simulink model "defaultCtrlModel"  (R2022a)
settings: Solver=FixedStepAuto  StartTime=0.0  StopTime=1800  FixedStep=Ts  RelTol=1e-3
values from neighbouring files (symbols this model uses):
  Kt = 0.882355004501468    (= 0.882355004501)    [initModels_GUI.m]
  N = 3.75    [compareAdmittance.m]    (also in initModels_GUI.m)
libraries: simulink x2
settings Model: Creator=Johannes  LastModifiedBy=Johannes
settings SolverCC: ConcurrentTasks=on  AlgebraicLoopSolver=TrustRegion  PositivePriorityOrder=on
settings OptimizationCC: BlockReduction=off  OptimizeBlockIOStorage=off  ZeroExternalMemoryAtStartup=off  ZeroInternalMemoryAtStartup=off
settings DebuggingCC: TasksWithSamePriorityMsg=none  UnconnectedInputMsg=warning  UnconnectedOutputMsg=warning  UnconnectedLineMsg=warning  SFMachineParentedDataDiag=warning
settings HardwareCC: ProdBitPerLong=64  ProdLongLongMode=on  ProdHWDeviceType=Intel->x86-64 (Linux 64)
settings RTWCC: Description=Generic Real-Time Target  Toolchain=Simulink Real-Time Toolchain  BuildConfiguration=Faster Runs  TargetLang=C++  DLArmComputeVersion=19.05
settings GRTTargetCC: TargetLangStandard=C++03 (ISO)  CodeInterfacePackaging=C++ class

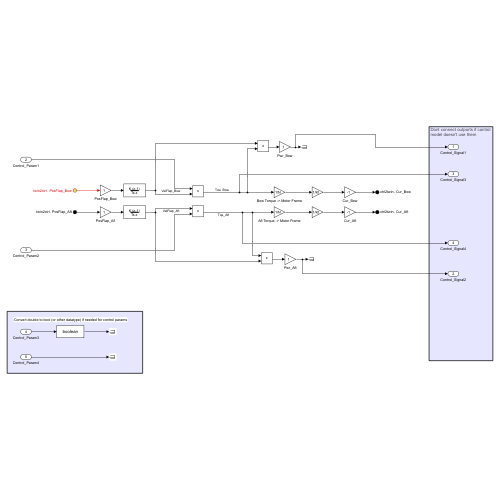
[thumbnail: Simulink's stored preview of the top-level diagram]
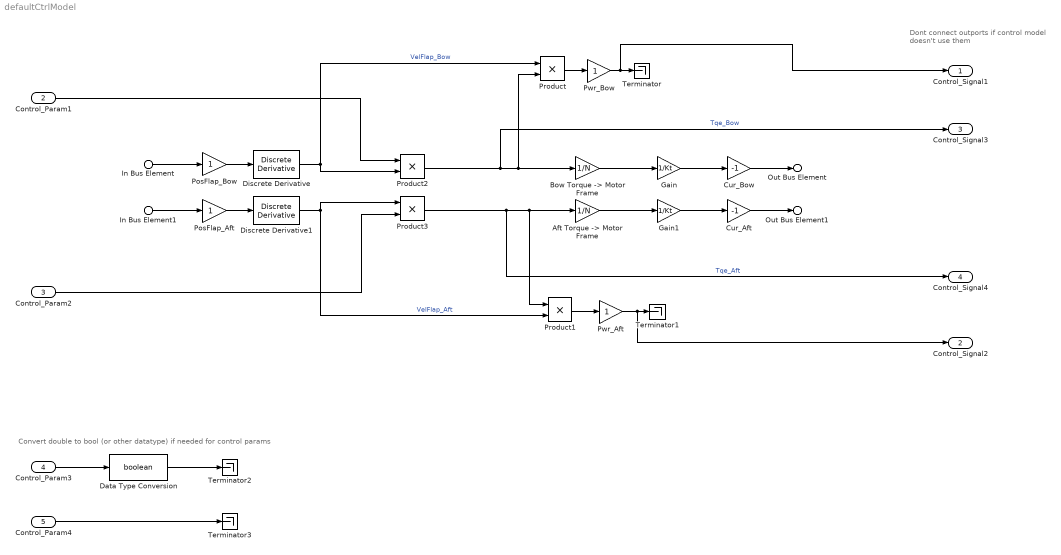
== system defaultCtrlModel ==
  note: Dont connect outports if control
      | model doesn't use them
  note: Convert double to bool (or other datatype) if needed for control params
  In Bus Element : Inport  PortName=twin2ctrl  Element=PosFlap_Bow
  In Bus Element1 : Inport  PortName=twin2ctrl  Element=PosFlap_Aft
  Control_Param1 : Inport  Port=2
  Control_Param2 : Inport  Port=3
  Control_Param3 : Inport  Port=4  OutDataTypeStr=double
  Control_Param4 : Inport  Port=5  OutDataTypeStr=double
  "Aft Torque -> Motor Frame" : Gain  Gain=1/N
  "Bow Torque -> Motor Frame" : Gain  Gain=1/N
  Cur_Aft : Gain  Gain=-1
  Cur_Bow : Gain  Gain=-1
  Data Type Conversion : DataTypeConversion  OutDataTypeStr=boolean  SaturateOnIntegerOverflow=off  RndMeth=Floor
  Discrete Derivative : simulink/Discrete/Discrete Derivative  gainval=1.0  ICPrevScaledInput=0.0  OutMin=[]  OutMax=[]  OutDataType=fixdt(1, 16)  OutScaling=2^-10  DoSatur=off
  Discrete Derivative1 : simulink/Discrete/Discrete Derivative  gainval=1.0  ICPrevScaledInput=0.0  OutMin=[]  OutMax=[]  OutDataType=fixdt(1, 16)  OutScaling=2^-10  DoSatur=off
  Gain : Gain  Gain=1/Kt
  Gain1 : Gain  Gain=1/Kt
  PosFlap_Aft : Gain
  PosFlap_Bow : Gain
  Product{,1..3} (4 alike) : Product
  Pwr_Aft : Gain
  Pwr_Bow : Gain
  Terminator{,1..3} (4 alike) : Terminator
  Control_Signal1 : Outport
  Control_Signal2 : Outport  Port=2
  Control_Signal3 : Outport  Port=3
  Control_Signal4 : Outport  Port=4
  Out Bus Element : Outport  Port=5  PortName=ctrl2twin  Element=Cur_Bow
  Out Bus Element1 : Outport  Port=5  PortName=ctrl2twin  Element=Cur_Aft
  wires:
  PosFlap_Bow/1 -> Discrete Derivative/1
  Discrete Derivative/1 -> Product/1, Product2/2  "VelFlap_Bow"
  Product3/1 -> Control_Signal4/1, "Aft Torque -> Motor Frame"/1, Product1/1  "Tqe_Aft"
  In Bus Element/1 -> PosFlap_Bow/1
  Discrete Derivative1/1 -> Product3/1, Product1/2  "VelFlap_Aft"
  Cur_Bow/1 -> Out Bus Element/1
  Cur_Aft/1 -> Out Bus Element1/1
  In Bus Element1/1 -> PosFlap_Aft/1
  Gain1/1 -> Cur_Aft/1
  Product1/1 -> Pwr_Aft/1
  Pwr_Aft/1 -> Control_Signal2/1, Terminator1/1
  Product/1 -> Pwr_Bow/1
  Gain/1 -> Cur_Bow/1
  PosFlap_Aft/1 -> Discrete Derivative1/1
  Product2/1 -> Control_Signal3/1, "Bow Torque -> Motor Frame"/1, Product/2  "Tqe_Bow"
  Pwr_Bow/1 -> Control_Signal1/1, Terminator/1
  Control_Param2/1 -> Product3/2
  Control_Param1/1 -> Product2/1
  Control_Param3/1 -> Data Type Conversion/1
  Data Type Conversion/1 -> Terminator2/1
  Control_Param4/1 -> Terminator3/1
  "Bow Torque -> Motor Frame"/1 -> Gain/1
  "Aft Torque -> Motor Frame"/1 -> Gain1/1
